simulink model "Lab2_Simulink_Design_Part3_2"  (R2020a)
settings: Solver=VariableStepAuto  StartTime=0.0  StopTime=10.0  RelTol=1e-3
settings Model: Creator=mati1  LastModifiedBy=mati1

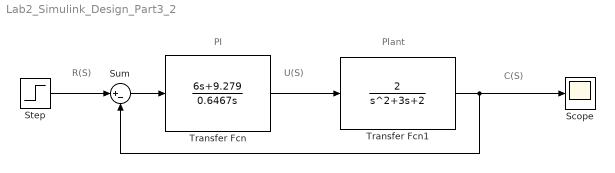
== system Lab2_Simulink_Design_Part3_2 ==
  note: R(S)
  note: C(S)
  note: U(S)
  note: Plant
  note: PI
  Scope : Scope
  Step : Step  Before=1  SampleTime=0
  Sum : Sum  Inputs=|+-
  Transfer Fcn : TransferFcn  Numerator=[6 9.279]  Denominator=[0.6467 0]
  Transfer Fcn1 : TransferFcn  Numerator=[2]  Denominator=[1 3 2]
  wires:
  Sum/1 -> Transfer Fcn/1
  Step/1 -> Sum/1
  Transfer Fcn1/1 -> Scope/1, Sum/2
  Transfer Fcn/1 -> Transfer Fcn1/1
